simulink model "controlador"  (R2015a)
settings: Solver=ode45  StartTime=0.0  StopTime=20  RelTol=1e-3
values from neighbouring files (symbols this model uses):
  A = A    [design.m]    (also in init.mat = [2.98564337206 1 0 0 0 -3.00327796547 0 1 0 0 0.709627661926)
  B = B    [design.m]    (also in init.mat = [1 0 0 0 0])
  D = zeros(1+length(A(:,1)),1)    [design.m]    (also in init.mat = 0)
  H = [C;eye(size(A))]    [design.m]
undefined symbols (not defined in the file or in its folder): K
settings Model: Creator=João  LastModifiedBy=João

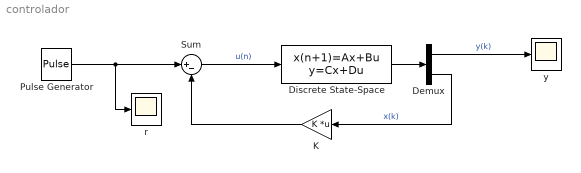
== system controlador ==
  Demux : Demux  Outputs=2
  Discrete State-Space : DiscreteStateSpace  A=A  B=B  C=H  D=D  SampleTime=0.02
  K : Gain  Gain=K  Multiplication=Matrix(K*u) (u vector)
  Pulse Generator : DiscretePulseGenerator  PulseType=Time based  Period=20  PhaseDelay=2
  Sum : Sum  Inputs=|+-
  r : Scope
      settings: SaveName=r_c  SampleInput=on
  y : Scope
      settings: SaveName=y_c  SampleInput=on
  wires:
  Sum/1 -> Discrete State-Space/1  "u(n)"
  Discrete State-Space/1 -> Demux/1
  Demux/2 -> K/1  "x(k)"
  Pulse Generator/1 -> Sum/1, r/1
  K/1 -> Sum/2
  Demux/1 -> y/1  "y(k)"
